simulink model "kinem_simu"  (R2025b)
settings: Solver=VariableStepAuto  StartTime=0.0  StopTime=10.0  RelTol=1e-3
libraries: simulink x1
settings Model: Creator=schar  LastModifiedBy=schar

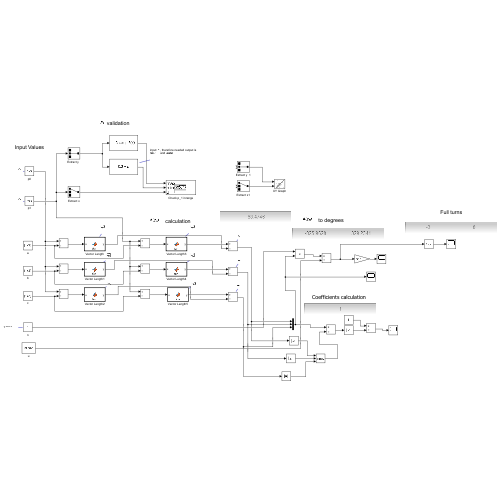
[thumbnail: Simulink's stored preview of the top-level diagram]
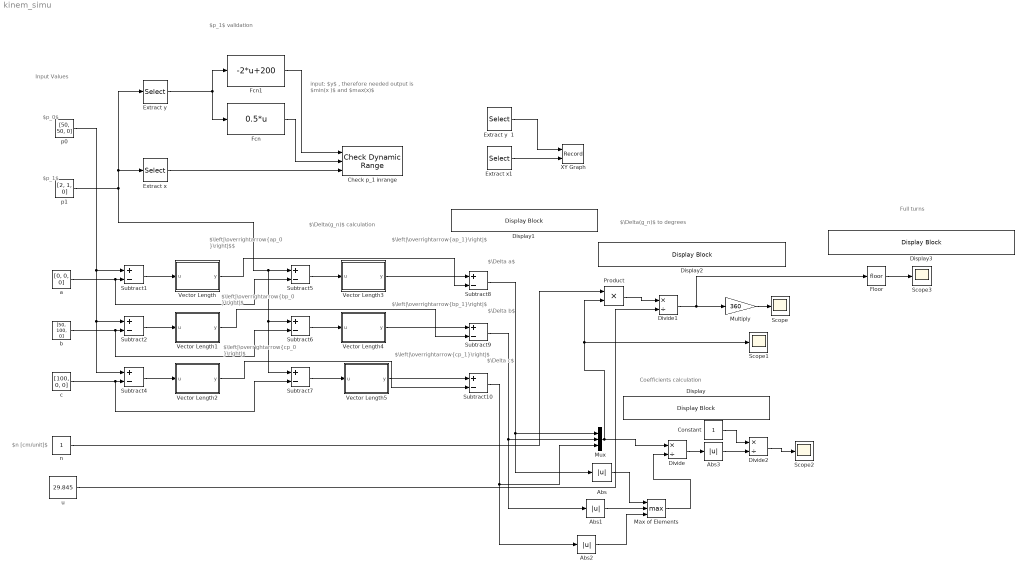
== system kinem_simu ==
  note: $n [cm/unit]$
  note: Coefficients calculation
  note: Input Values
  note: $p_1$ validation
  note: $\Delta(g_n)$ calculation
  note: $\Delta a$
  note: $\left|\overrightarrow{ap_0 }\right|$$
  note: $p_1$
  note: input: $y$ , therefore needed output is $min(x )$ and $max(x)$
  note: $p_0$
  note: $\left|\overrightarrow{bp_0 }\right|$
  note: $\left|\overrightarrow{cp_0 }\right|$
  note: $\left|\overrightarrow{cp_1}\right|$
  note: $\left|\overrightarrow{bp_1}\right|$
  note: $\left|\overrightarrow{ap_1}\right|$
  note: $\Delta b$
  note: $\Delta c$
  note: $\Delta(g_n)$ to degrees
  note: Full turns
  Abs{,1..3} (4 alike) : Abs  SaturateOnIntegerOverflow=off
  Check p_1 inrange : simulink/Model Verification/Check  Dynamic Range  Description=min < u < max  enabled=on  stopWhenAssertionFail=on  export=off  icon=graphic
  Constant : Constant
  Display{,1..3} (4 alike) : DisplayBlock  LabelPosition=Hide  Transparency=1  GridColor=[0.502, 0.502, 0.502]
  Divide : Product  Inputs=*/
  Divide1 : Product  Inputs=*/
  Divide2 : Product  Inputs=*/
  Extract x : Selector  InputPortWidth=3  IndexOptions=Index vector (dialog)  Indices=[1]  OutputSizes=1
  Extract x1 : Selector  InputPortWidth=3  IndexOptions=Index vector (dialog)  Indices=[1]  OutputSizes=1
  "Extract y  " : Selector  InputPortWidth=3  IndexOptions=Index vector (dialog)  Indices=[2]  OutputSizes=1
  Extract y  1 : Selector  InputPortWidth=3  IndexOptions=Index vector (dialog)  Indices=[2]  OutputSizes=1
  Fcn : Fcn  Expr=0.5*u
  Fcn1 : Fcn  Expr=-2*u+200
  Floor : Rounding
  Max of Elements : MinMax  Function=max  Inputs=3
  Multiply : Gain  Gain=360
  Mux : Mux  Inputs=3
  Product : Product
  Scope{,1..3} (4 alike) : Scope
      Scope settings: ActiveDisplayYMinimum=-1231.860688198653  ActiveDisplayYMaximum=1265.1909364490421
      Scope1 settings: ActiveDisplayYMinimum=-177.01253425895334  ActiveDisplayYMaximum=147.75805967343746  DataLoggingVariableName=ScopeData2
      Scope2 settings: ActiveDisplayYMinimum=27.431875330559716  ActiveDisplayYMaximum=98.0059305479397
      Scope3 settings: DataLoggingVariableName=ScopeData3
  Subtract{1..2,4..10} (9 alike) : Sum  Inputs=+-
  Vector Length : MATLAB Function  TreatAsAtomicUnit=on
  Vector Length1 : MATLAB Function  TreatAsAtomicUnit=on
  Vector Length2 : MATLAB Function  TreatAsAtomicUnit=on
  Vector Length3 : MATLAB Function  TreatAsAtomicUnit=on
  Vector Length4 : MATLAB Function  TreatAsAtomicUnit=on
  Vector Length5 : MATLAB Function  TreatAsAtomicUnit=on
  XY Graph : Record  NumPorts=2.0  FileSettingsInternal="{\"entries\":[{\"content\":{\"excelSettings\":{\"content\":{},\"type\":\"Streamout.ExcelSettings\"},\"parquetSettings\":{\"content\":{},\"type\":\"Streamout.ParquetSettings\"}},\"type\":\"Streamout.FileSettingStorage\",\"uuid\":\"\"}],\"packageUris\":[\"http:\\/\\/schema.mathworks.com\\/mf0\\/streamout_blocks\\/R2020a\"],\"version\":\"1.0\"}"  FrameSettings=[0, 0]  Layout=[1 1]  SignalsInternal="{\"entries\":[{\"content\":{\"signals\":[{\"content\":{\"blockPath\":[],\"dimensions\":[1],\"domain\":\"\",\"lineColor\":\"#a2142f\",\"plots\":[ 1 ],\"port\":1,\"sid\":[\"\"],\"signalID\":1,\"signalName\":\"Extract y  1\"},\"type\":\"RecordBlkView.Signal\",\"uuid\":\"\"},{\"content\":{\"blockPath\":[],\"dimensions\":[1],\"domain\":\"\",\"lineColor\":\"#139fff\",\"plots\":[ 1 ],\"port\":2,\"sid\":[\"\"],\"signalID\":2,\"signalName\":\"Extract x1\"},\"type\":\"RecordBlkView.Signal\",\"uuid\":\"\"}]},\"type\":\"RecordBlkView.InputSignals\",\"uuid\":\"\"}],\"packageUris\":[\"http:\\/\\/schema.mathworks.com\\/mf0\\/streamout_blocks\\/R2020a\"],\"version\":\"1.0\"}"  VisualizationBindings="{\"xyplotplugin\":{\"info\":[{\"series\":[{\"bindingParametersList\":[{\"parameter\":\"X-Axis\",\"signalID\":1,\"signalName\":\"Extract y  1\"},{\"parameter\":\"Y-Axis\",\"signalID\":2,\"signalName\":\"Extract x1\"}],\"seriesID\":0}],\"subplotID\":1}]}}"  CompatibilityTag=XY
  a : Constant  Value=[0, 0, 0]
  b : Constant  Value=[50, 100, 0]
  c : Constant  Value=[100, 0, 0]
  n : Constant
  p0 : Constant  Value=[50, 50, 0]
  p1 : Constant  Value=[2, 1, 0]
  u : Constant  Value=29.845
  wires:
  Extract x/1 -> Check p_1 inrange/3
  p1/1 -> Subtract5/1, Subtract6/1, Subtract7/1, "Extract y  "/1, Extract x/1
  "Extract y  "/1 -> Fcn1/1, Fcn/1
  Fcn/1 -> Check p_1 inrange/2
  Fcn1/1 -> Check p_1 inrange/1
  Extract y  1/1 -> XY Graph/1
  Extract x1/1 -> XY Graph/2
  p0/1 -> Subtract4/1, Subtract2/1, Subtract1/1
  a/1 -> Subtract5/2, Subtract1/2
  b/1 -> Subtract6/2, Subtract2/2
  c/1 -> Subtract7/2, Subtract4/2
  Subtract1/1 -> Vector Length/1(u)
  Subtract2/1 -> Vector Length1/1(u)
  Subtract4/1 -> Vector Length2/1(u)
  Subtract7/1 -> Vector Length5/1(u)
  Subtract5/1 -> Vector Length3/1(u)
  Subtract6/1 -> Vector Length4/1(u)
  Vector Length/1(y) -> Subtract8/2
  Vector Length1/1(y) -> Subtract9/2
  Vector Length2/1(y) -> Subtract10/2
  Subtract8/1 -> Mux/1, Abs/1
  Subtract10/1 -> Mux/3, Abs2/1
  Subtract9/1 -> Mux/2, Abs1/1
  Vector Length3/1(y) -> Subtract8/1
  Vector Length4/1(y) -> Subtract9/1
  Vector Length5/1(y) -> Subtract10/1
  Abs/1 -> Max of Elements/1
  Abs1/1 -> Max of Elements/2
  Abs2/1 -> Max of Elements/3
  Max of Elements/1 -> Divide/2
  Mux/1 -> Product/2, Scope1/1, Divide/1
  Divide/1 -> Abs3/1
  n/1 -> Product/1
  Product/1 -> Divide1/1
  u/1 -> Divide1/2
  Divide1/1 -> Floor/1, Multiply/1
  Multiply/1 -> Scope/1
  Floor/1 -> Scope3/1
  Constant/1 -> Divide2/1
  Abs3/1 -> Divide2/2
  Divide2/1 -> Scope2/1

== matlab function kinem_simu/Vector Length1 ==
  data: u input; y output
function y = fcn(u)

y = norm(u);

== matlab function kinem_simu/Vector Length2 ==
  data: u input; y output
function y = fcn(u)

y = norm(u);

== matlab function kinem_simu/Vector Length3 ==
  data: u input; y output
function y = fcn(u)

y = norm(u);

== matlab function kinem_simu/Vector Length4 ==
  data: u input; y output
function y = fcn(u)

y = norm(u);

== matlab function kinem_simu/Vector Length5 ==
  data: u input; y output
function y = fcn(u)

y = norm(u);

== matlab function kinem_simu/Vector Length ==
  data: u input; y output
function y = fcn(u)

y = norm(u);
